simulink model "TST_EGRVlv_DDSens"  (R2016b)
settings: Solver=FixedStepDiscrete  StartTime=0.0  StopTime=simTime  FixedStep=sampleTime  RelTol=1e-3
values from neighbouring files (symbols this model uses):
  testCase = 1    [initTST_EGRVlv_DDSens_001.m]
libraries: simulink x11, UnitTest_Lib x9
settings Model: Creator=zhengjinyan  LastModifiedBy=zhengjinyan
settings DebuggingCC: SignalRangeChecking=error

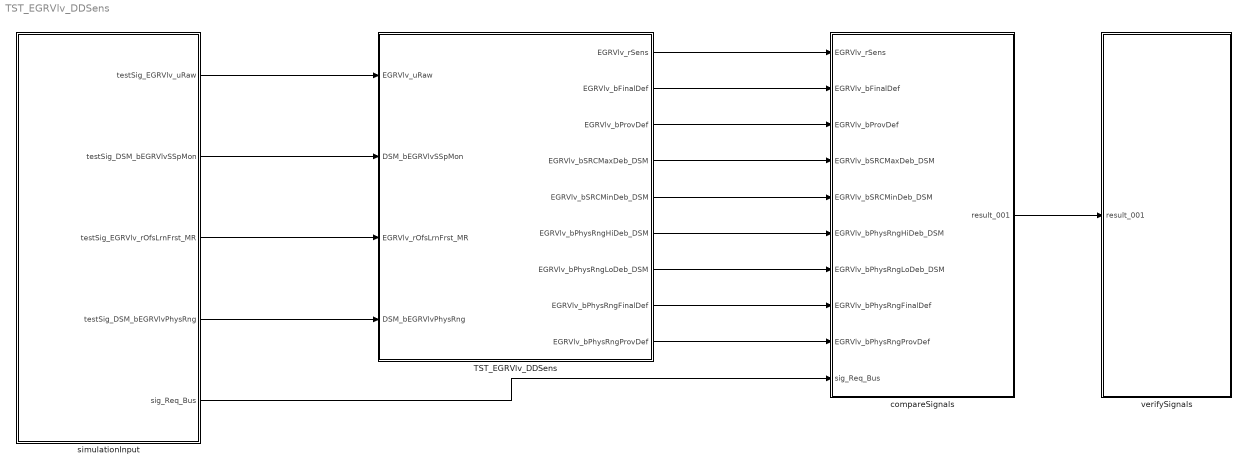
== system TST_EGRVlv_DDSens ==
  TST_EGRVlv_DDSens : Subsystem
  compareSignals : Subsystem
  simulationInput : Subsystem
  verifySignals : Subsystem
  wires:
  simulationInput/1(testSig_EGRVlv_uRaw) -> TST_EGRVlv_DDSens/1(EGRVlv_uRaw)
  simulationInput/2(testSig_DSM_bEGRVlvSSpMon) -> TST_EGRVlv_DDSens/2(DSM_bEGRVlvSSpMon)
  simulationInput/3(testSig_EGRVlv_rOfsLrnFrst_MR) -> TST_EGRVlv_DDSens/3(EGRVlv_rOfsLrnFrst_MR)
  simulationInput/4(testSig_DSM_bEGRVlvPhysRng) -> TST_EGRVlv_DDSens/4(DSM_bEGRVlvPhysRng)
  TST_EGRVlv_DDSens/1(EGRVlv_rSens) -> compareSignals/1(EGRVlv_rSens)
  TST_EGRVlv_DDSens/2(EGRVlv_bFinalDef) -> compareSignals/2(EGRVlv_bFinalDef)
  TST_EGRVlv_DDSens/3(EGRVlv_bProvDef) -> compareSignals/3(EGRVlv_bProvDef)
  TST_EGRVlv_DDSens/4(EGRVlv_bSRCMaxDeb_DSM) -> compareSignals/4(EGRVlv_bSRCMaxDeb_DSM)
  TST_EGRVlv_DDSens/5(EGRVlv_bSRCMinDeb_DSM) -> compareSignals/5(EGRVlv_bSRCMinDeb_DSM)
  TST_EGRVlv_DDSens/6(EGRVlv_bPhysRngHiDeb_DSM) -> compareSignals/6(EGRVlv_bPhysRngHiDeb_DSM)
  TST_EGRVlv_DDSens/7(EGRVlv_bPhysRngLoDeb_DSM) -> compareSignals/7(EGRVlv_bPhysRngLoDeb_DSM)
  TST_EGRVlv_DDSens/8(EGRVlv_bPhysRngFinalDef) -> compareSignals/8(EGRVlv_bPhysRngFinalDef)
  TST_EGRVlv_DDSens/9(EGRVlv_bPhysRngProvDef) -> compareSignals/9(EGRVlv_bPhysRngProvDef)
  simulationInput/5(sig_Req_Bus) -> compareSignals/10(sig_Req_Bus)
  compareSignals/1(result_001) -> verifySignals/1(result_001)

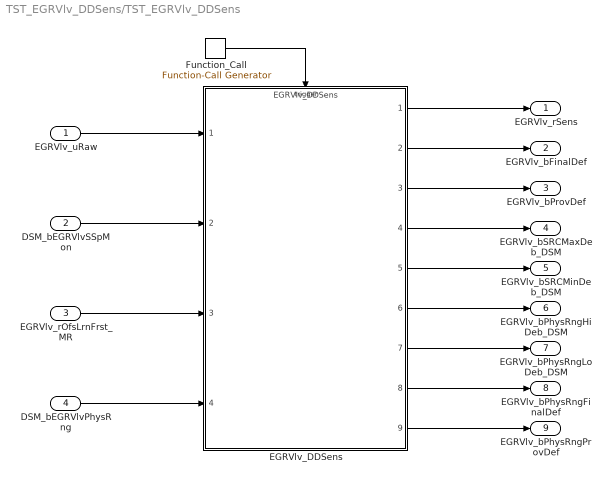
== system TST_EGRVlv_DDSens/TST_EGRVlv_DDSens ==
  EGRVlv_uRaw : Inport
  DSM_bEGRVlvSSpMon : Inport  Port=2
  EGRVlv_rOfsLrnFrst_MR : Inport  Port=3
  DSM_bEGRVlvPhysRng : Inport  Port=4
  EGRVlv_DDSens : ModelReference  ModelNameDialog=EGRVlv_DDSens  SimulationMode=Normal  ModelReferenceVersion=1.13  TriggerPortName=function  TriggerPortTriggerType=function-call  TriggerPortStatesWhenEnabling=held
  Function_Call : simulink/Ports & Subsystems/Function-Call Generator  sample_time=sampleTime  numberOfIterations=1
  EGRVlv_rSens : Outport
  EGRVlv_bFinalDef : Outport  Port=2
  EGRVlv_bProvDef : Outport  Port=3
  EGRVlv_bSRCMaxDeb_DSM : Outport  Port=4
  EGRVlv_bSRCMinDeb_DSM : Outport  Port=5
  EGRVlv_bPhysRngHiDeb_DSM : Outport  Port=6
  EGRVlv_bPhysRngLoDeb_DSM : Outport  Port=7
  EGRVlv_bPhysRngFinalDef : Outport  Port=8
  EGRVlv_bPhysRngProvDef : Outport  Port=9
  wires:
  Function_Call/1 -> EGRVlv_DDSens/Trigger
  EGRVlv_uRaw/1 -> EGRVlv_DDSens/1
  DSM_bEGRVlvSSpMon/1 -> EGRVlv_DDSens/2
  EGRVlv_rOfsLrnFrst_MR/1 -> EGRVlv_DDSens/3
  DSM_bEGRVlvPhysRng/1 -> EGRVlv_DDSens/4
  EGRVlv_DDSens/1 -> EGRVlv_rSens/1
  EGRVlv_DDSens/2 -> EGRVlv_bFinalDef/1
  EGRVlv_DDSens/3 -> EGRVlv_bProvDef/1
  EGRVlv_DDSens/4 -> EGRVlv_bSRCMaxDeb_DSM/1
  EGRVlv_DDSens/5 -> EGRVlv_bSRCMinDeb_DSM/1
  EGRVlv_DDSens/6 -> EGRVlv_bPhysRngHiDeb_DSM/1
  EGRVlv_DDSens/7 -> EGRVlv_bPhysRngLoDeb_DSM/1
  EGRVlv_DDSens/8 -> EGRVlv_bPhysRngFinalDef/1
  EGRVlv_DDSens/9 -> EGRVlv_bPhysRngProvDef/1

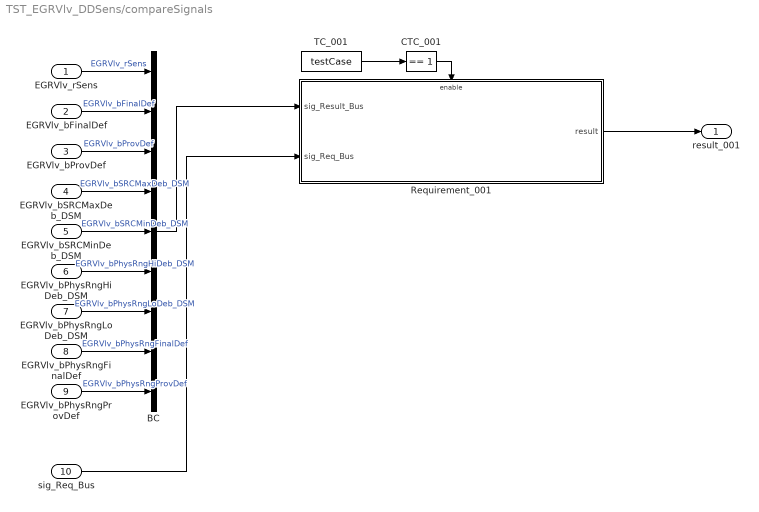
== system TST_EGRVlv_DDSens/compareSignals ==
  EGRVlv_rSens : Inport
  EGRVlv_bFinalDef : Inport  Port=2
  EGRVlv_bProvDef : Inport  Port=3
  EGRVlv_bSRCMaxDeb_DSM : Inport  Port=4
  EGRVlv_bSRCMinDeb_DSM : Inport  Port=5
  EGRVlv_bPhysRngHiDeb_DSM : Inport  Port=6
  EGRVlv_bPhysRngLoDeb_DSM : Inport  Port=7
  EGRVlv_bPhysRngFinalDef : Inport  Port=8
  EGRVlv_bPhysRngProvDef : Inport  Port=9
  sig_Req_Bus : Inport  Port=10
  BC : BusCreator  Inputs=9
  CTC_001 : simulink/Logic and Bit Operations/Compare To Constant  relop===  const=1  OutDataTypeStr=boolean
  Requirement_001 : Subsystem
  TC_001 : Constant  Value=testCase
  result_001 : Outport
  wires:
  EGRVlv_rSens/1 -> BC/1  "EGRVlv_rSens"
  EGRVlv_bFinalDef/1 -> BC/2  "EGRVlv_bFinalDef"
  EGRVlv_bProvDef/1 -> BC/3  "EGRVlv_bProvDef"
  EGRVlv_bSRCMaxDeb_DSM/1 -> BC/4  "EGRVlv_bSRCMaxDeb_DSM"
  EGRVlv_bSRCMinDeb_DSM/1 -> BC/5  "EGRVlv_bSRCMinDeb_DSM"
  EGRVlv_bPhysRngHiDeb_DSM/1 -> BC/6  "EGRVlv_bPhysRngHiDeb_DSM"
  EGRVlv_bPhysRngLoDeb_DSM/1 -> BC/7  "EGRVlv_bPhysRngLoDeb_DSM"
  EGRVlv_bPhysRngFinalDef/1 -> BC/8  "EGRVlv_bPhysRngFinalDef"
  EGRVlv_bPhysRngProvDef/1 -> BC/9  "EGRVlv_bPhysRngProvDef"
  TC_001/1 -> CTC_001/1
  CTC_001/1 -> Requirement_001/Enable
  sig_Req_Bus/1 -> Requirement_001/2(sig_Req_Bus)
  BC/1 -> Requirement_001/1(sig_Result_Bus)
  Requirement_001/1(result) -> result_001/1

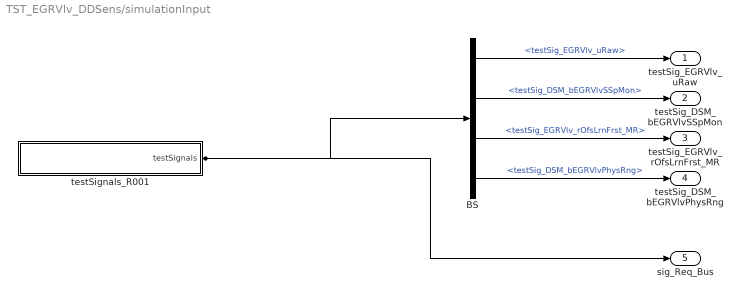
== system TST_EGRVlv_DDSens/simulationInput ==
  BS : BusSelector  OutputSignals=testSig_EGRVlv_uRaw,testSig_DSM_bEGRVlvSSpMon,testSig_EGRVlv_rOfsLrnFrst_MR,testSig_DSM_bEGRVlvPhysRng
  testSignals_R001 : Subsystem
  testSig_EGRVlv_uRaw : Outport
  testSig_DSM_bEGRVlvSSpMon : Outport  Port=2
  testSig_EGRVlv_rOfsLrnFrst_MR : Outport  Port=3
  testSig_DSM_bEGRVlvPhysRng : Outport  Port=4
  sig_Req_Bus : Outport  Port=5
  wires:
  BS/1 -> testSig_EGRVlv_uRaw/1  "<testSig_EGRVlv_uRaw>"
  BS/2 -> testSig_DSM_bEGRVlvSSpMon/1  "<testSig_DSM_bEGRVlvSSpMon>"
  BS/3 -> testSig_EGRVlv_rOfsLrnFrst_MR/1  "<testSig_EGRVlv_rOfsLrnFrst_MR>"
  BS/4 -> testSig_DSM_bEGRVlvPhysRng/1  "<testSig_DSM_bEGRVlvPhysRng>"
  testSignals_R001/1(testSignals) -> BS/1, sig_Req_Bus/1

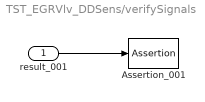
== system TST_EGRVlv_DDSens/verifySignals ==
  result_001 : Inport
  Assertion_001 : Assertion  Enabled=off
  wires:
  result_001/1 -> Assertion_001/1

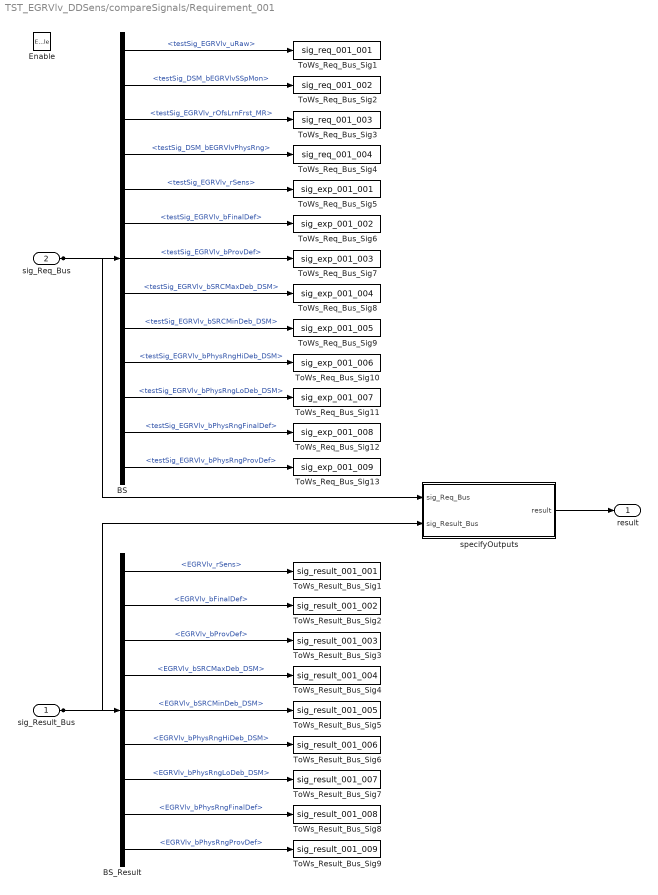
== system TST_EGRVlv_DDSens/compareSignals/Requirement_001 ==
  sig_Result_Bus : Inport
  sig_Req_Bus : Inport  Port=2
  Enable : EnablePort
  BS : BusSelector  OutputSignals=testSig_EGRVlv_uRaw,testSig_DSM_bEGRVlvSSpMon,testSig_EGRVlv_rOfsLrnFrst_MR,testSig_DSM_bEGRVlvPhysRng,testSig_EGRVlv_rSens,testSig_EGRVlv_bFinalDef,testSig_EGRVlv_bProvDef,testSig_EGRVlv_bSRCMaxDeb_DSM,testSig_EGRVlv_bSRCMinDeb_DSM,testSig_EGRVlv_bPhysRngHiDeb_DSM,testSig_EGRVlv_bPhysRngLoDeb_DSM,testSig_EGRVlv_bPhysRngFinalDef,testSig_EGRVlv_bPhysRngProvDef
  BS_Result : BusSelector  OutputSignals=EGRVlv_rSens,EGRVlv_bFinalDef,EGRVlv_bProvDef,EGRVlv_bSRCMaxDeb_DSM,EGRVlv_bSRCMinDeb_DSM,EGRVlv_bPhysRngHiDeb_DSM,EGRVlv_bPhysRngLoDeb_DSM,EGRVlv_bPhysRngFinalDef,EGRVlv_bPhysRngProvDef
  ToWs_Req_Bus_Sig1 : ToWorkspace  VariableName=sig_req_001_001  SaveFormat=Structure With Time
  ToWs_Req_Bus_Sig10 : ToWorkspace  VariableName=sig_exp_001_006  SaveFormat=Structure With Time
  ToWs_Req_Bus_Sig11 : ToWorkspace  VariableName=sig_exp_001_007  SaveFormat=Structure With Time
  ToWs_Req_Bus_Sig12 : ToWorkspace  VariableName=sig_exp_001_008  SaveFormat=Structure With Time
  ToWs_Req_Bus_Sig13 : ToWorkspace  VariableName=sig_exp_001_009  SaveFormat=Structure With Time
  ToWs_Req_Bus_Sig2 : ToWorkspace  VariableName=sig_req_001_002  SaveFormat=Structure With Time
  ToWs_Req_Bus_Sig3 : ToWorkspace  VariableName=sig_req_001_003  SaveFormat=Structure With Time
  ToWs_Req_Bus_Sig4 : ToWorkspace  VariableName=sig_req_001_004  SaveFormat=Structure With Time
  ToWs_Req_Bus_Sig5 : ToWorkspace  VariableName=sig_exp_001_001  SaveFormat=Structure With Time
  ToWs_Req_Bus_Sig6 : ToWorkspace  VariableName=sig_exp_001_002  SaveFormat=Structure With Time
  ToWs_Req_Bus_Sig7 : ToWorkspace  VariableName=sig_exp_001_003  SaveFormat=Structure With Time
  ToWs_Req_Bus_Sig8 : ToWorkspace  VariableName=sig_exp_001_004  SaveFormat=Structure With Time
  ToWs_Req_Bus_Sig9 : ToWorkspace  VariableName=sig_exp_001_005  SaveFormat=Structure With Time
  ToWs_Result_Bus_Sig1 : ToWorkspace  VariableName=sig_result_001_001  SaveFormat=Structure With Time
  ToWs_Result_Bus_Sig2 : ToWorkspace  VariableName=sig_result_001_002  SaveFormat=Structure With Time
  ToWs_Result_Bus_Sig3 : ToWorkspace  VariableName=sig_result_001_003  SaveFormat=Structure With Time
  ToWs_Result_Bus_Sig4 : ToWorkspace  VariableName=sig_result_001_004  SaveFormat=Structure With Time
  ToWs_Result_Bus_Sig5 : ToWorkspace  VariableName=sig_result_001_005  SaveFormat=Structure With Time
  ToWs_Result_Bus_Sig6 : ToWorkspace  VariableName=sig_result_001_006  SaveFormat=Structure With Time
  ToWs_Result_Bus_Sig7 : ToWorkspace  VariableName=sig_result_001_007  SaveFormat=Structure With Time
  ToWs_Result_Bus_Sig8 : ToWorkspace  VariableName=sig_result_001_008  SaveFormat=Structure With Time
  ToWs_Result_Bus_Sig9 : ToWorkspace  VariableName=sig_result_001_009  SaveFormat=Structure With Time
  specifyOutputs : Subsystem
  result : Outport
  wires:
  sig_Req_Bus/1 -> BS/1, specifyOutputs/1(sig_Req_Bus)
  BS/1 -> ToWs_Req_Bus_Sig1/1  "<testSig_EGRVlv_uRaw>"
  BS/2 -> ToWs_Req_Bus_Sig2/1  "<testSig_DSM_bEGRVlvSSpMon>"
  BS/3 -> ToWs_Req_Bus_Sig3/1  "<testSig_EGRVlv_rOfsLrnFrst_MR>"
  BS/4 -> ToWs_Req_Bus_Sig4/1  "<testSig_DSM_bEGRVlvPhysRng>"
  BS/5 -> ToWs_Req_Bus_Sig5/1  "<testSig_EGRVlv_rSens>"
  BS/6 -> ToWs_Req_Bus_Sig6/1  "<testSig_EGRVlv_bFinalDef>"
  BS/7 -> ToWs_Req_Bus_Sig7/1  "<testSig_EGRVlv_bProvDef>"
  BS/8 -> ToWs_Req_Bus_Sig8/1  "<testSig_EGRVlv_bSRCMaxDeb_DSM>"
  BS/9 -> ToWs_Req_Bus_Sig9/1  "<testSig_EGRVlv_bSRCMinDeb_DSM>"
  BS/10 -> ToWs_Req_Bus_Sig10/1  "<testSig_EGRVlv_bPhysRngHiDeb_DSM>"
  BS/11 -> ToWs_Req_Bus_Sig11/1  "<testSig_EGRVlv_bPhysRngLoDeb_DSM>"
  BS/12 -> ToWs_Req_Bus_Sig12/1  "<testSig_EGRVlv_bPhysRngFinalDef>"
  BS/13 -> ToWs_Req_Bus_Sig13/1  "<testSig_EGRVlv_bPhysRngProvDef>"
  sig_Result_Bus/1 -> BS_Result/1, specifyOutputs/2(sig_Result_Bus)
  BS_Result/1 -> ToWs_Result_Bus_Sig1/1  "<EGRVlv_rSens>"
  BS_Result/2 -> ToWs_Result_Bus_Sig2/1  "<EGRVlv_bFinalDef>"
  BS_Result/3 -> ToWs_Result_Bus_Sig3/1  "<EGRVlv_bProvDef>"
  BS_Result/4 -> ToWs_Result_Bus_Sig4/1  "<EGRVlv_bSRCMaxDeb_DSM>"
  BS_Result/5 -> ToWs_Result_Bus_Sig5/1  "<EGRVlv_bSRCMinDeb_DSM>"
  BS_Result/6 -> ToWs_Result_Bus_Sig6/1  "<EGRVlv_bPhysRngHiDeb_DSM>"
  BS_Result/7 -> ToWs_Result_Bus_Sig7/1  "<EGRVlv_bPhysRngLoDeb_DSM>"
  BS_Result/8 -> ToWs_Result_Bus_Sig8/1  "<EGRVlv_bPhysRngFinalDef>"
  BS_Result/9 -> ToWs_Result_Bus_Sig9/1  "<EGRVlv_bPhysRngProvDef>"
  specifyOutputs/1(result) -> result/1

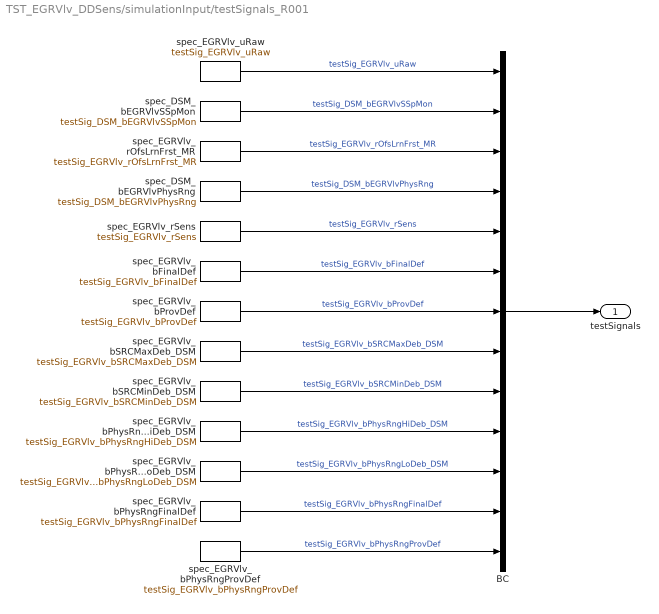
== system TST_EGRVlv_DDSens/simulationInput/testSignals_R001 ==
  BC : BusCreator  Inputs=13
  spec_DSM_bEGRVlvPhysRng : FromWorkspace  VariableName=testSig_DSM_bEGRVlvPhysRng  Interpolate=off  OutputAfterFinalValue=Holding final value
  spec_DSM_bEGRVlvSSpMon : FromWorkspace  VariableName=testSig_DSM_bEGRVlvSSpMon  Interpolate=off  OutputAfterFinalValue=Holding final value
  spec_EGRVlv_bFinalDef : FromWorkspace  VariableName=testSig_EGRVlv_bFinalDef  Interpolate=off  OutputAfterFinalValue=Holding final value
  spec_EGRVlv_bPhysRngFinalDef : FromWorkspace  VariableName=testSig_EGRVlv_bPhysRngFinalDef  Interpolate=off  OutputAfterFinalValue=Holding final value
  spec_EGRVlv_bPhysRngHiDeb_DSM : FromWorkspace  VariableName=testSig_EGRVlv_bPhysRngHiDeb_DSM  Interpolate=off  OutputAfterFinalValue=Holding final value
  spec_EGRVlv_bPhysRngLoDeb_DSM : FromWorkspace  VariableName=testSig_EGRVlv_bPhysRngLoDeb_DSM  Interpolate=off  OutputAfterFinalValue=Holding final value
  spec_EGRVlv_bPhysRngProvDef : FromWorkspace  VariableName=testSig_EGRVlv_bPhysRngProvDef  Interpolate=off  OutputAfterFinalValue=Holding final value
  spec_EGRVlv_bProvDef : FromWorkspace  VariableName=testSig_EGRVlv_bProvDef  Interpolate=off  OutputAfterFinalValue=Holding final value
  spec_EGRVlv_bSRCMaxDeb_DSM : FromWorkspace  VariableName=testSig_EGRVlv_bSRCMaxDeb_DSM  Interpolate=off  OutputAfterFinalValue=Holding final value
  spec_EGRVlv_bSRCMinDeb_DSM : FromWorkspace  VariableName=testSig_EGRVlv_bSRCMinDeb_DSM  Interpolate=off  OutputAfterFinalValue=Holding final value
  spec_EGRVlv_rOfsLrnFrst_MR : FromWorkspace  VariableName=testSig_EGRVlv_rOfsLrnFrst_MR  Interpolate=off  OutputAfterFinalValue=Holding final value
  spec_EGRVlv_rSens : FromWorkspace  VariableName=testSig_EGRVlv_rSens  Interpolate=off  OutputAfterFinalValue=Holding final value
  spec_EGRVlv_uRaw : FromWorkspace  VariableName=testSig_EGRVlv_uRaw  Interpolate=off  OutputAfterFinalValue=Holding final value
  testSignals : Outport
  wires:
  BC/1 -> testSignals/1
  spec_EGRVlv_uRaw/1 -> BC/1  "testSig_EGRVlv_uRaw"
  spec_DSM_bEGRVlvSSpMon/1 -> BC/2  "testSig_DSM_bEGRVlvSSpMon"
  spec_EGRVlv_rOfsLrnFrst_MR/1 -> BC/3  "testSig_EGRVlv_rOfsLrnFrst_MR"
  spec_DSM_bEGRVlvPhysRng/1 -> BC/4  "testSig_DSM_bEGRVlvPhysRng"
  spec_EGRVlv_rSens/1 -> BC/5  "testSig_EGRVlv_rSens"
  spec_EGRVlv_bFinalDef/1 -> BC/6  "testSig_EGRVlv_bFinalDef"
  spec_EGRVlv_bProvDef/1 -> BC/7  "testSig_EGRVlv_bProvDef"
  spec_EGRVlv_bSRCMaxDeb_DSM/1 -> BC/8  "testSig_EGRVlv_bSRCMaxDeb_DSM"
  spec_EGRVlv_bSRCMinDeb_DSM/1 -> BC/9  "testSig_EGRVlv_bSRCMinDeb_DSM"
  spec_EGRVlv_bPhysRngHiDeb_DSM/1 -> BC/10  "testSig_EGRVlv_bPhysRngHiDeb_DSM"
  spec_EGRVlv_bPhysRngLoDeb_DSM/1 -> BC/11  "testSig_EGRVlv_bPhysRngLoDeb_DSM"
  spec_EGRVlv_bPhysRngFinalDef/1 -> BC/12  "testSig_EGRVlv_bPhysRngFinalDef"
  spec_EGRVlv_bPhysRngProvDef/1 -> BC/13  "testSig_EGRVlv_bPhysRngProvDef"

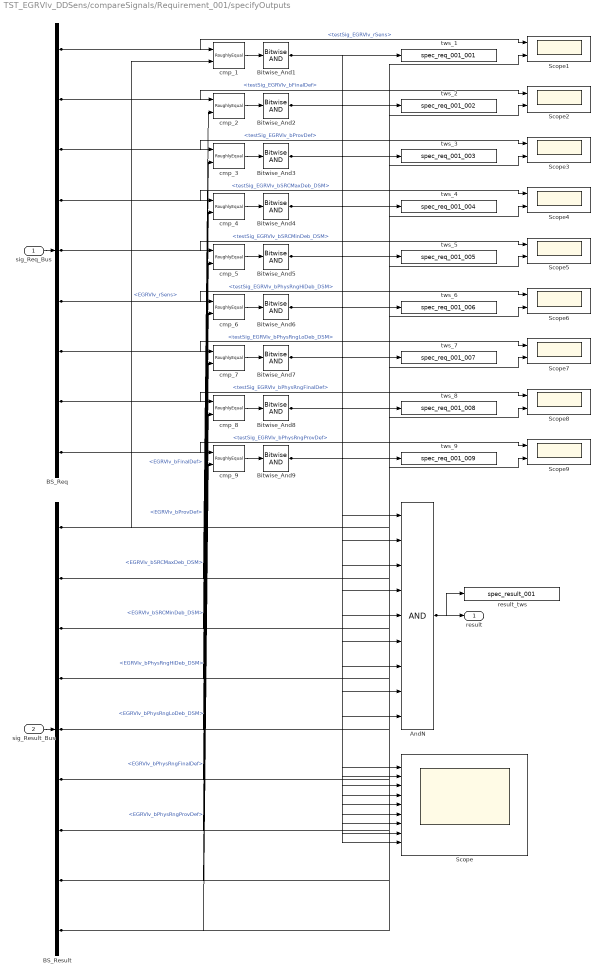
== system TST_EGRVlv_DDSens/compareSignals/Requirement_001/specifyOutputs ==
  sig_Req_Bus : Inport
  sig_Result_Bus : Inport  Port=2
  AndN : Logic  Inputs=9
  BS_Req : BusSelector  OutputSignals=testSig_EGRVlv_rSens,testSig_EGRVlv_bFinalDef,testSig_EGRVlv_bProvDef,testSig_EGRVlv_bSRCMaxDeb_DSM,testSig_EGRVlv_bSRCMinDeb_DSM,testSig_EGRVlv_bPhysRngHiDeb_DSM,testSig_EGRVlv_bPhysRngLoDeb_DSM,testSig_EGRVlv_bPhysRngFinalDef,testSig_EGRVlv_bPhysRngProvDef
  BS_Result : BusSelector  OutputSignals=EGRVlv_rSens,EGRVlv_bFinalDef,EGRVlv_bProvDef,EGRVlv_bSRCMaxDeb_DSM,EGRVlv_bSRCMinDeb_DSM,EGRVlv_bPhysRngHiDeb_DSM,EGRVlv_bPhysRngLoDeb_DSM,EGRVlv_bPhysRngFinalDef,EGRVlv_bPhysRngProvDef
  Bitwise_And{1..9} (9 alike) : simulink/Logic and Bit Operations/Bitwise Operator  logicop=AND  UseBitMask=off  BitMask=bin2dec('11011001')  BitMaskRealWorld=Stored Integer
  Scope : Scope  NumInputPorts=9
  Scope{1..9} (9 alike) : Scope  NumInputPorts=2
  cmp_{1..9} (9 alike) : UnitTest_Lib/RoughlyEqual  slope=0.1
  result_tws : ToWorkspace  VariableName=spec_result_001
  tws_1 : ToWorkspace  VariableName=spec_req_001_001
  tws_2 : ToWorkspace  VariableName=spec_req_001_002
  tws_3 : ToWorkspace  VariableName=spec_req_001_003
  tws_4 : ToWorkspace  VariableName=spec_req_001_004
  tws_5 : ToWorkspace  VariableName=spec_req_001_005
  tws_6 : ToWorkspace  VariableName=spec_req_001_006
  tws_7 : ToWorkspace  VariableName=spec_req_001_007
  tws_8 : ToWorkspace  VariableName=spec_req_001_008
  tws_9 : ToWorkspace  VariableName=spec_req_001_009
  result : Outport
  wires:
  sig_Req_Bus/1 -> BS_Req/1
  sig_Result_Bus/1 -> BS_Result/1
  AndN/1 -> result/1, result_tws/1
  BS_Req/1 -> cmp_1/1, Scope1/1  "<testSig_EGRVlv_rSens>"
  BS_Result/1 -> cmp_1/2, Scope1/2  "<EGRVlv_rSens>"
  cmp_1/1 -> Bitwise_And1/1
  Bitwise_And1/1 -> tws_1/1, AndN/1, Scope/1
  BS_Req/2 -> cmp_2/1, Scope2/1  "<testSig_EGRVlv_bFinalDef>"
  BS_Result/2 -> cmp_2/2, Scope2/2  "<EGRVlv_bFinalDef>"
  cmp_2/1 -> Bitwise_And2/1
  Bitwise_And2/1 -> tws_2/1, AndN/2, Scope/2
  BS_Req/3 -> cmp_3/1, Scope3/1  "<testSig_EGRVlv_bProvDef>"
  BS_Result/3 -> cmp_3/2, Scope3/2  "<EGRVlv_bProvDef>"
  cmp_3/1 -> Bitwise_And3/1
  Bitwise_And3/1 -> tws_3/1, AndN/3, Scope/3
  BS_Req/4 -> cmp_4/1, Scope4/1  "<testSig_EGRVlv_bSRCMaxDeb_DSM>"
  BS_Result/4 -> cmp_4/2, Scope4/2  "<EGRVlv_bSRCMaxDeb_DSM>"
  cmp_4/1 -> Bitwise_And4/1
  Bitwise_And4/1 -> tws_4/1, AndN/4, Scope/4
  BS_Req/5 -> cmp_5/1, Scope5/1  "<testSig_EGRVlv_bSRCMinDeb_DSM>"
  BS_Result/5 -> cmp_5/2, Scope5/2  "<EGRVlv_bSRCMinDeb_DSM>"
  cmp_5/1 -> Bitwise_And5/1
  Bitwise_And5/1 -> tws_5/1, AndN/5, Scope/5
  BS_Req/6 -> cmp_6/1, Scope6/1  "<testSig_EGRVlv_bPhysRngHiDeb_DSM>"
  BS_Result/6 -> cmp_6/2, Scope6/2  "<EGRVlv_bPhysRngHiDeb_DSM>"
  cmp_6/1 -> Bitwise_And6/1
  Bitwise_And6/1 -> tws_6/1, AndN/6, Scope/6
  BS_Req/7 -> cmp_7/1, Scope7/1  "<testSig_EGRVlv_bPhysRngLoDeb_DSM>"
  BS_Result/7 -> cmp_7/2, Scope7/2  "<EGRVlv_bPhysRngLoDeb_DSM>"
  cmp_7/1 -> Bitwise_And7/1
  Bitwise_And7/1 -> tws_7/1, AndN/7, Scope/7
  BS_Req/8 -> cmp_8/1, Scope8/1  "<testSig_EGRVlv_bPhysRngFinalDef>"
  BS_Result/8 -> cmp_8/2, Scope8/2  "<EGRVlv_bPhysRngFinalDef>"
  cmp_8/1 -> Bitwise_And8/1
  Bitwise_And8/1 -> tws_8/1, AndN/8, Scope/8
  BS_Req/9 -> cmp_9/1, Scope9/1  "<testSig_EGRVlv_bPhysRngProvDef>"
  BS_Result/9 -> cmp_9/2, Scope9/2  "<EGRVlv_bPhysRngProvDef>"
  cmp_9/1 -> Bitwise_And9/1
  Bitwise_And9/1 -> tws_9/1, AndN/9, Scope/9
